simulink model "Exercitiul_2"  (R2021b)
settings: Solver=VariableStepAuto  StartTime=0.0  StopTime=10.0  RelTol=1e-3
values from neighbouring files (symbols this model uses):
  A_c = double(A_c)    [Exercitiul_1.m]
  A_o = double(A_o)    [Exercitiul_1.m]
  B_c = double(B_c)    [Exercitiul_1.m]
  B_o = double(B_o)    [Exercitiul_1.m]
  C_c = double(C_c)    [Exercitiul_1.m]
  C_o = double(C_o)    [Exercitiul_1.m]
  D_c = [0 0]    [Exercitiul_1.m]
  D_o = [0 0]    [Exercitiul_1.m]
settings Model: Creator=edwar  LastModifiedBy=edwar

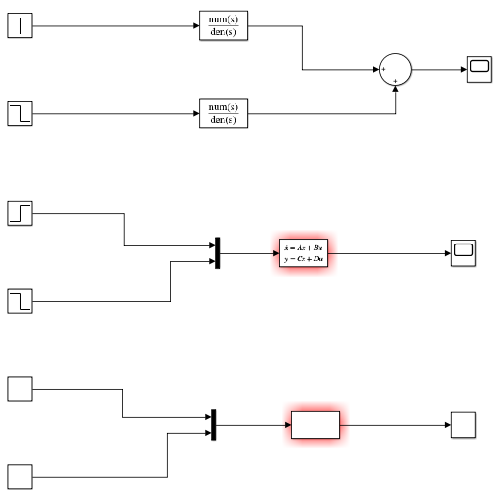
[thumbnail: Simulink's stored preview of the top-level diagram]
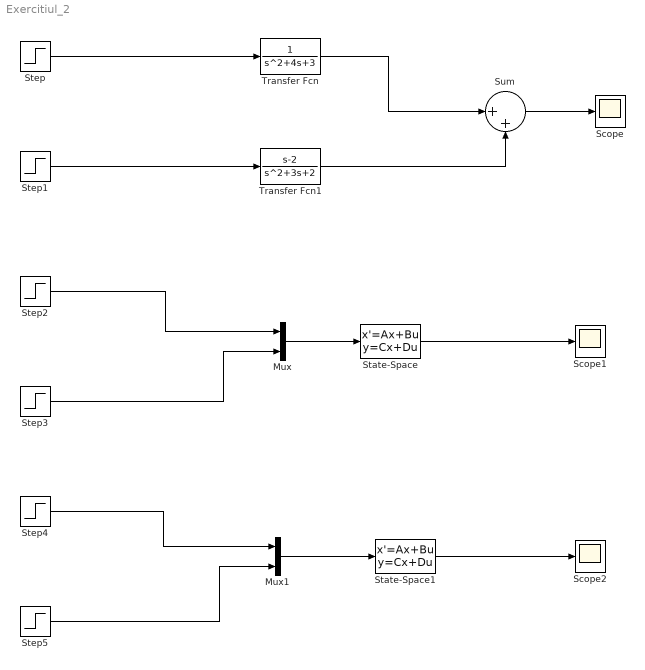
== system Exercitiul_2 ==
  Mux : Mux  Inputs=2
  Mux1 : Mux  Inputs=2
  Scope : Scope
  Scope1 : Scope
  Scope2 : Scope
  State-Space : StateSpace  A=A_c  B=B_c  C=C_c  D=D_c  InitialCondition=0
  State-Space1 : StateSpace  A=A_o  B=B_o  C=C_o  D=D_o  InitialCondition=0
  Step : Step  Time=0  SampleTime=0
  Step1 : Step  Time=0  After=-2  SampleTime=0
  Step2 : Step  Time=0  SampleTime=0
  Step3 : Step  Time=0  After=-2  SampleTime=0
  Step4 : Step  Time=0  SampleTime=0
  Step5 : Step  Time=0  After=-2  SampleTime=0
  Sum : Sum  Inputs=|++
  Transfer Fcn : TransferFcn  Numerator=1  Denominator=[1 4 3]
  Transfer Fcn1 : TransferFcn  Numerator=[1 -2]  Denominator=[1 3 2]
  wires:
  Transfer Fcn/1 -> Sum/1
  Step4/1 -> Mux1/1
  Mux1/1 -> State-Space1/1
  Step1/1 -> Transfer Fcn1/1
  Sum/1 -> Scope/1
  State-Space/1 -> Scope1/1
  Step2/1 -> Mux/1
  Mux/1 -> State-Space/1
  Step5/1 -> Mux1/2
  Transfer Fcn1/1 -> Sum/2
  Step/1 -> Transfer Fcn/1
  State-Space1/1 -> Scope2/1
  Step3/1 -> Mux/2
